simulink model "SISO_FullstateFeedbackDesign"  (R2025b)
settings: Solver=VariableStepAuto  StartTime=0.0  StopTime=40  RelTol=1e-3
undefined symbols (not defined in the file or in its folder): linmodel, op
libraries: eeLuenbergerObserver x1, Drone_SISO_Subsystem x1
settings Model: Creator=Alek  LastModifiedBy=Alek

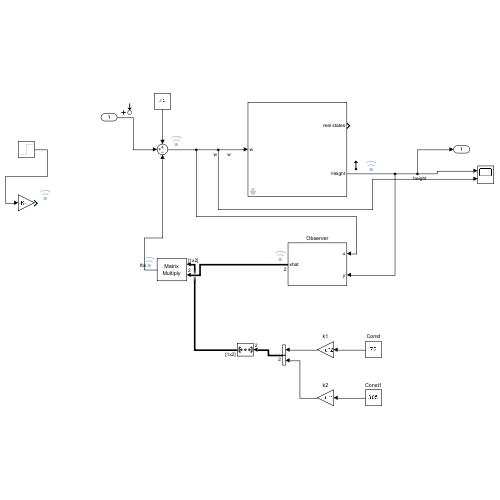
[thumbnail: Simulink's stored preview of the top-level diagram]
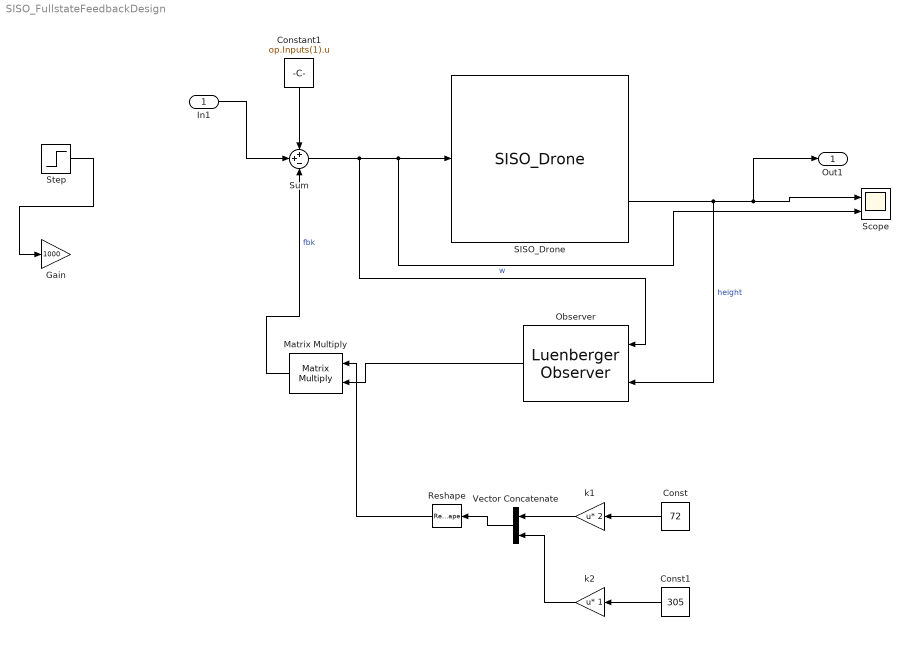
== system SISO_FullstateFeedbackDesign ==
  In1 : Inport
  Const : Constant  Value=72
  Const1 : Constant  Value=305
  Constant1 : Constant  Value=op.Inputs(1).u
  Gain : Gain  Gain=1000
  Matrix Multiply : Product  Multiplication=Matrix(*)
  Observer : eeLuenbergerObserver/Luenberger Observer  StateSpaceType=Continuous-time  Ad=1  Bd=1  Cd=1  Dd=1  A=linmodel.A  B=linmodel.B  C=linmodel.C  D=linmodel.D  ObserverDesign=Desired eigenvalues  Ld=1  DesiredEigenvalues=[-150+400j -150-400j]  x0=[0; 0]  Tsd=0.001  Ts=0.005
      settings: LibrarySourceBlock=ee_sl_lib/Observers/Luenberger Observer
  Reshape : Reshape  OutputDimensionality=Row vector (2-D)
  SISO_Drone : Drone_SISO_Subsystem/SISO_Drone  kf=1e-5  m=0.5  l=1e-2  I=6.6666e-5
      settings: SourceProductName=Drone SISO Plant
  Scope : Scope  NumInputPorts=2
      settings: ActiveDisplayYMinimum=-5858.4071531181926  ActiveDisplayYMaximum=3522.6581859097782
  Step : Step  Time=0  SampleTime=0
  Sum : Sum  Inputs=++-
  Vector Concatenate : Concatenate
  k1 : Gain  Gain=2  Multiplication=Matrix(u*K)
  k2 : Gain  Multiplication=Matrix(u*K)
  Out1 : Outport
  wires:
  SISO_Drone/2 -> Observer/2, Out1/1, Scope/1  "height"
  Step/1 -> Gain/1
  Sum/1 -> Observer/1, Scope/2, SISO_Drone/1  "w"
  Observer/1 -> Matrix Multiply/2
  Matrix Multiply/1 -> Sum/3  "fbk"
  Constant1/1 -> Sum/1
  In1/1 -> Sum/2
  Const/1 -> k1/1
  Reshape/1 -> Matrix Multiply/1
  k1/1 -> Vector Concatenate/1
  Vector Concatenate/1 -> Reshape/1
  k2/1 -> Vector Concatenate/2
  Const1/1 -> k2/1
